simulink model "MicroMouseTemplate"  (R2024a)
settings: Solver=FixedStepAuto  StartTime=0.0  StopTime=2  RelTol=1e-3  EnableMultiTasking=on
undefined symbols (not defined in the file): samplingTime
settings Model: STM32="{\"DigitalPortWrite\":[{\"ID\":\"MicroMouseTemplate:84:3\"},{\"ID\":\"MicroMouseTemplate:84:4\"},{\"ID\":\"MicroMouseTemplate:84:5\"},{\"ID\":\"MicroMouseTemplate:84:6\"},{\"ID\":\"MicroMouseTemplate:84:7\"},{\"ID\":\"MicroMouseTemplate:84:8\"},{\"ID\":\"MicroMouseTemplate:84:9\"},{\"ID\":\"MicroMouseTemplate:84:10\"},{\"ID\":\"MicroMouseTemplate:160:19\"},{\"ID\":\"MicroMouseTemplate:2479:4\"},{\"ID\":\"MicroMouseTemplate:2479:6\"},{\"ID\":\"MicroMouseTemplate:2479:7\"},{\"ID\":\"MicroMouseTemplate:2479:8\"},{\"ID\":\"MicroMouseTemplate1:84:3\"},{\"ID\":\"MicroMouseTemplate1:84:4\"},{\"ID\":\"MicroMouseTemplate1:84:5\"},{\"ID\":\"MicroMouseTemplate1:84:6\"},{\"ID\":\"MicroMouseTemplate1:84:7\"},{\"ID\":\"MicroMouseTemplate1:84:8\"},{\"ID\":\"MicroMouseTemplate1:84:9\"},{\"ID\":\"MicroMouseTemplate1:84:10\"},{\"ID\":\"MicroMouseTemplate1:160:19\"},{\"ID\":\"MicroMouseTemplate1:2479:4\"},{\"ID\":\"MicroMouseTemplate1:2479:6\"},{\"ID\":\"MicroMouseTemplate1:2479:7\"},{\"ID\":\"MicroMouseTemplate1:2479:8\"}],\"PWMOutput\":[{\"ID\":\"MicroMouseTemplate:160:24\"},{\"ID\":\"MicroMouseTemplate:160:25\"},{\"ID\":\"MicroMouseTemplate1:160:24\"},{\"ID\":\"MicroMouseTemplate1:160:25\"}],\"AnalogInput\":[{\"ID\":\"MicroMouseTemplate:2357:1\"},{\"ID\":\"MicroMouseTemplate1:2357:1\"}],\"DigitalPortRead\":[{\"ID\":\"MicroMouseTemplate:2483:3\"},{\"ID\":\"MicroMouseTemplate:2483:4\"},{\"ID\":\"MicroMouseTemplate1:2483:3\"},{\"ID\":\"MicroMouseTemplate1:2483:4\"}]}"  SimulationMode=external  ExtModeTrigDuration=10  Creator=JesseJabezArendse  LastModifiedBy=phila
settings SolverCC: AllowMultiTaskInputOutput=on  AutoInsertRateTranBlk=on  InsertRTBMode=Never (minimum delay)
settings OptimizationCC: EnhancedBackFolding=on  PassReuseOutputArgsAs=Individual arguments  StateBitsets=on  DataBitsets=on  ZeroExternalMemoryAtStartup=off  ZeroInternalMemoryAtStartup=off  NoFixptDivByZeroProtection=on  MaxStackSize=64  OptimizeBlockOrder=speed  DifferentSizesBufferReuse=on  EfficientTunableParamExpr=on
settings DebuggingCC: MultiTaskCondExecSysMsg=none  ParameterOverflowMsg=none  ParameterPrecisionLossMsg=none  ParameterTunabilityLossMsg=error
settings HardwareCC: ProdBitPerPointer=32  ProdBitPerSizeT=32  ProdBitPerPtrDiffT=32  ProdLargestAtomicInteger=Long  ProdLargestAtomicFloat=Double  ProdWordSize=32  ProdLongLongMode=on  ProdHWDeviceType=ARM Compatible->ARM Cortex  TargetBitPerPointer=64  TargetBitPerSizeT=64  TargetBitPerPtrDiffT=64  TargetLongLongMode=on  TargetIntDivRoundTo=Zero  TargetEndianess=LittleEndian  TargetWordSize=64  TargetHWDeviceType=MATLAB Host
settings ModelReferenceCC: EnableParallelModelReferenceBuilds=on  ParallelModelReferenceMATLABWorkerInit=Copy Base Workspace  SupportModelReferenceSimTargetCustomCode=on
settings SFSimCC: MATLABDynamicMemAlloc=off  SimHardwareAcceleration=native
settings RTWCC: Description=Embedded Coder  SystemTargetFile=ert.tlc  HardwareBoard=STM32L4xx Based  TLCOptions=-p0 -aInlineSetEventsForThisBaseRateFcn=TLC_FALSE -aSuppressMultiTaskScheduler=TLC_FALSE -aRateBasedStepFcn=1  TemplateMakefile=ert_default_tmf  Toolchain=GNU Tools for ARM Embedded Processors  CodeExecutionProfiling=on  CodeProfilingInstrumentation=coarse  GPUComputeCapability=3.5
settings RTWCC: CustomHeaderCode=|
  | #include "MicroMouseProgramming\Core\Inc\IMU.h"
  | #include "MicroMouseProgramming\Core\Inc\CustomWhile.h"
  | #include "MicroMouseProgramming\Core\Inc\Motors.h"
settings RTWCC: CustomInclude=|
  | MicroMouseProgramming\Core\Inc\
  | MicroMouseProgramming\Core\Src\
settings RTWCC: CustomSource=|
  | MicroMouseProgramming\Core\Src\IMU.c
  | MicroMouseProgramming\Core\Src\CustomWhile.c
  | MicroMouseProgramming\Core\Src\Motors.c
settings CodeAppCC: ForceParamTrailComments=on  IgnoreCustomStorageClasses=off  OperatorAnnotations=on  SimulinkDataObjDesc=on  SFDataObjDesc=on  InsertBlockDesc=on
settings ERTTargetCC: CodeReplacementLibrary=ARM Cortex-M  SupportNonFinite=off  SupportComplex=off  ExtModeTransport=3  ExtModeStaticAlloc=on  ExtModeStaticAllocSize=2048  ExtModeMexFile=ext_xcp  ExtModeIntrfLevel=Level2 - Open

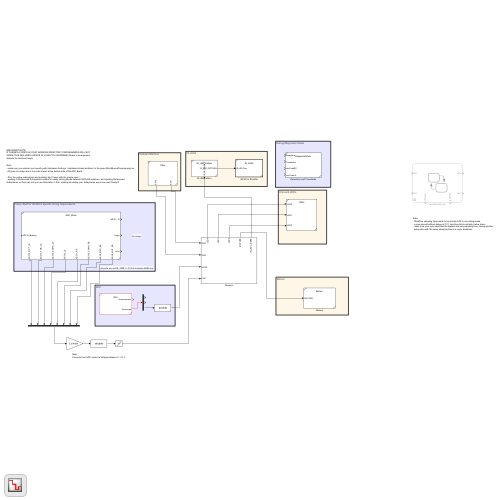
[thumbnail: Simulink's stored preview of the top-level diagram]
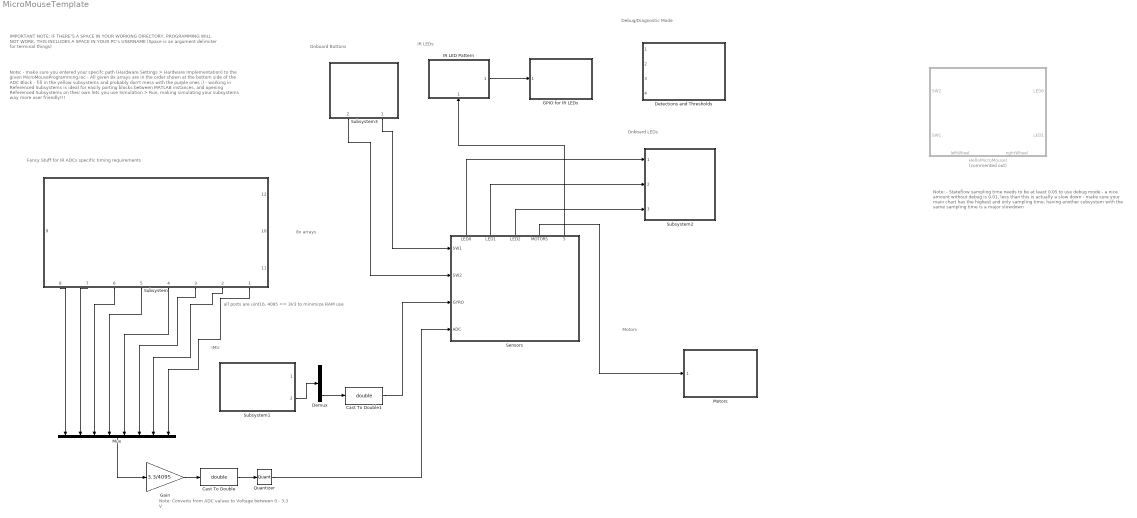
== system MicroMouseTemplate ==
  note: IMPORTANT NOTE:
      | IF THERE'S A SPACE IN YOUR WORKING DIRECTORY, PROGRAMMING WILL NOT WORK, THIS INCLUDES A SPACE IN YOUR PC's USERNAME (Space is an argument delimiter for terminal things)
  note: Note:
      | - make sure you entered your specifc path (Hardware Settings > Hardware Implementation) to the given MicroMouseProgramming.ioc
      | - All given 8x arrays are in the order shown at the bottom side of the ADC Block
      |
      | - fill in the yellow subsystems and probably don't mess with the purple ones :)
      | - working in Referenced Subsystems is ideal for easily porting blocks between MATLAB instances, and opening Referenced Subsystems on their own lets you use Simulation > Run, making simulating your subsystems way more user friendly!!!
  note: 8x arrays
  note: all ports are uint16, 4095 == 3V3 to minimize RAM use
  note: IMU
  note: Note:
      | - Stateflow sampling time needs to be at least 0.05 to use debug mode
      | - a nice amount without debug is 0.01, less than this is actually a slow down
      | - make sure your main chart has the highest and only sampling time, having another
      | subsystem with the same sampling time is a major slowdown
  note: Fancy Stuff for IR ADCs specific timing requirements
  note: IR LEDs
  note: Motors
  note: Onboard Buttons
  note: Onboard LEDs
  note: Debug/Diagnostic Mode
  note: Note:
      | Converts from ADC values to Voltage between 0 - 3.3 V
  Cast To Double : DataTypeConversion  OutDataTypeStr=double  SaturateOnIntegerOverflow=off  RndMeth=Floor
  Cast To Double1 : DataTypeConversion  OutDataTypeStr=double  SaturateOnIntegerOverflow=off  RndMeth=Floor
  Demux : Demux  Outputs=3
  Detections and Thresholds : Subsystem  ReferencedSubsystem=DiagnosticMode
  GPIO for IR LEDs : Subsystem  TreatAsAtomicUnit=on  SystemSampleTime=samplingTime  ReferencedSubsystem=IR_LEDs
  Gain : Gain  Gain=3.3/4095
  HelloMicroMouse! : Stateflow chart  Commented=on  TreatAsAtomicUnit=on
      settings: PortSchema="{\"entries\":[{\"content\":{\"sides\":[{\"content\":{\"connectorIds\":[\"In1\",\"In2\"]},\"type\":\"ConnectorPlacement.EquallySpacedRectSide\",\"uuid\":\"f52daa4f-6374-42e5-9ef1-0ccc99d09b58\"},{\"content\":{\"connectorIds\":[\"Out1\",\"Out2\"],\"side\":\"RIGHT\"},\"type\":\"ConnectorPlacement.EquallySpacedRectSide\",\"uuid\":\"94b478cc-4dde-45c7-a588-77cf2b43cdb7\"},{\"content\":{\"side\":\"TOP\"},\"type\":\"ConnectorPlacement.EquallySpacedRectSide\",\"uuid\":\"afff2079-ea5c-423e-9722-09c3bbce433b\"},{\"content\":{\"connectorIds\":[\"Out3\",\"Out4\"],\"side\":\"BOTTOM\"},\"type\":\"ConnectorPlacement.EquallySpacedRectSide\",\"uuid\":\"94e93a1d-795d-41a3-b2d8-d520b2bf47ef\"}]},\"type\":\"ConnectorPlacement.EquallySpacedConnector\",\"uuid\":\"d4d35636-54af-48ac-af70-d56caef5e090\"}],\"packageUris\":[\"http://schema.mathworks.com/mf0/Connector/R2020b\"],\"version\":\"1.0\"}"
  IR LED Pattern : Subsystem  ReferencedSubsystem=IR_LED_Pattern
      settings: PortSchema="{\"entries\":[{\"content\":{\"sides\":[{\"content\":{},\"type\":\"ConnectorPlacement.EquallySpacedRectSide\",\"uuid\":\"7c8d8a80-aae0-409b-9cb9-b3b86d39018b\"},{\"content\":{\"connectorIds\":[\"Out1\"],\"side\":\"RIGHT\"},\"type\":\"ConnectorPlacement.EquallySpacedRectSide\",\"uuid\":\"c87144cc-2119-421f-99f2-b7a3c226c36e\"},{\"content\":{\"side\":\"TOP\"},\"type\":\"ConnectorPlacement.EquallySpacedRectSide\",\"uuid\":\"a76ebbaf-a86a-4c95-ac8a-0df310e45d39\"},{\"content\":{\"connectorIds\":[\"In1\"],\"side\":\"BOTTOM\"},\"type\":\"ConnectorPlacement.EquallySpacedRectSide\",\"uuid\":\"3df1aa50-ad1c-403c-a4a5-6da959ac349c\"}]},\"type\":\"ConnectorPlacement.EquallySpacedConnector\",\"uuid\":\"b655e760-2cb2-4645-8a40-e85195c99b66\"}],\"packageUris\":[\"http://schema.mathworks.com/mf0/Connector/R2020b\"],\"version\":\"1.0\"}"
  Motors : Subsystem  ReferencedSubsystem=Motors
  Mux : Mux  Inputs=8
  Quantizer : Quantizer  QuantizationInterval=0.01
  Sensors : Subsystem
      settings: PortSchema="{\"entries\":[{\"content\":{\"sides\":[{\"content\":{\"connectorIds\":[\"In1\",\"In2\",\"In3\",\"In4\"]},\"type\":\"ConnectorPlacement.EquallySpacedRectSide\",\"uuid\":\"bc6db5eb-46dc-4f8e-8cde-60f150010aca\"},{\"content\":{\"side\":\"RIGHT\"},\"type\":\"ConnectorPlacement.EquallySpacedRectSide\",\"uuid\":\"e71d750a-c6fe-4d02-b611-1eb45a9e699c\"},{\"content\":{\"connectorIds\":[\"Out1\",\"Out2\",\"Out3\",\"Out4\",\"Out5\"],\"side\":\"TOP\"},\"type\":\"ConnectorPlacement.EquallySpacedRectSide\",\"uuid\":\"16229a75-dc4c-4034-8ad6-a6d33f431b7e\"},{\"content\":{\"side\":\"BOTTOM\"},\"type\":\"ConnectorPlacement.EquallySpacedRectSide\",\"uuid\":\"378b0be1-cc28-458e-984c-d88580dc795a\"}]},\"type\":\"ConnectorPlacement.EquallySpacedConnector\",\"uuid\":\"81c8b409-cb86-489b-9c0e-9f4aaa37c54e\"}],\"packageUris\":[\"http://schema.mathworks.com/mf0/Connector/R2020b\"],\"version\":\"1.0\"}"
  Subsystem : Subsystem  ReferencedSubsystem=ADC_Block
      settings: PortSchema="{\"entries\":[{\"content\":{\"sides\":[{\"content\":{},\"type\":\"ConnectorPlacement.EquallySpacedRectSide\",\"uuid\":\"be6b81d5-7a49-4e34-b35f-0c07892094fc\"},{\"content\":{\"connectorIds\":[\"Out1\",\"Out2\",\"Out3\",\"Out4\",\"Out5\",\"Out6\",\"Out7\",\"Out8\"],\"side\":\"RIGHT\"},\"type\":\"ConnectorPlacement.EquallySpacedRectSide\",\"uuid\":\"5e22590a-b7c0-4c63-8de4-8d81fd6c3849\"},{\"content\":{\"connectorIds\":[\"Out12\",\"Out10\",\"Out11\"],\"side\":\"TOP\"},\"type\":\"ConnectorPlacement.EquallySpacedRectSide\",\"uuid\":\"da97636e-cea0-4a10-8fe5-d807f9ee999f\"},{\"content\":{\"connectorIds\":[\"Out9\"],\"side\":\"BOTTOM\"},\"type\":\"ConnectorPlacement.EquallySpacedRectSide\",\"uuid\":\"a593d780-81a8-4730-a8bc-2bbf356cafe4\"}]},\"type\":\"ConnectorPlacement.EquallySpacedConnector\",\"uuid\":\"0bcac921-e51a-4437-9183-315712d0a8c2\"}],\"packageUris\":[\"http://schema.mathworks.com/mf0/Connector/R2020b\"],\"version\":\"1.0\"}"
  Subsystem1 : Subsystem  ReferencedSubsystem=IMU
  Subsystem2 : Subsystem  ReferencedSubsystem=LEDs
  Subsystem3 : Subsystem  ReferencedSubsystem=SWs
      settings: PortSchema="{\"entries\":[{\"content\":{\"sides\":[{\"content\":{},\"type\":\"ConnectorPlacement.EquallySpacedRectSide\",\"uuid\":\"e28eebbe-b7f2-4b36-b777-f04b3fc0ab34\"},{\"content\":{\"side\":\"RIGHT\"},\"type\":\"ConnectorPlacement.EquallySpacedRectSide\",\"uuid\":\"8c3fa4f5-1e6a-4f41-8e39-119bdbcbe036\"},{\"content\":{\"side\":\"TOP\"},\"type\":\"ConnectorPlacement.EquallySpacedRectSide\",\"uuid\":\"44ec265b-fcc9-41a2-b2aa-224ec14b1e13\"},{\"content\":{\"connectorIds\":[\"Out2\",\"Out1\"],\"side\":\"BOTTOM\"},\"type\":\"ConnectorPlacement.EquallySpacedRectSide\",\"uuid\":\"b53c205f-8dfa-45db-b859-d3829686a648\"}]},\"type\":\"ConnectorPlacement.EquallySpacedConnector\",\"uuid\":\"83ae30f7-f6c1-458e-af88-9bb28644e581\"}],\"packageUris\":[\"http://schema.mathworks.com/mf0/Connector/R2020b\"],\"version\":\"1.0\"}"
  wires:
  IR LED Pattern/1 -> GPIO for IR LEDs/1
  Subsystem/2 -> Mux/7
  Subsystem/7 -> Mux/2
  Subsystem3/1 -> Sensors/1(SW1)
  Subsystem3/2 -> Sensors/2(SW2)
  Sensors/4(MOTORS) -> Motors/1
  Sensors/1(LED0) -> Subsystem2/1
  Subsystem/4 -> Mux/5
  Subsystem/5 -> Mux/4
  Subsystem/1 -> Mux/8
  Subsystem/3 -> Mux/6
  Subsystem/8 -> Mux/1
  Subsystem/6 -> Mux/3
  Quantizer/1 -> Sensors/4(ADC)
  Sensors/2(LED1) -> Subsystem2/2
  Sensors/3(LED2) -> Subsystem2/3
  Mux/1 -> Gain/1
  Cast To Double/1 -> Quantizer/1
  Gain/1 -> Cast To Double/1
  Sensors/5(IR_LEDs_SIDES) -> IR LED Pattern/1
  Demux/3 -> Cast To Double1/1
  Subsystem1/2 -> Demux/1
  Cast To Double1/1 -> Sensors/3(GYRO)

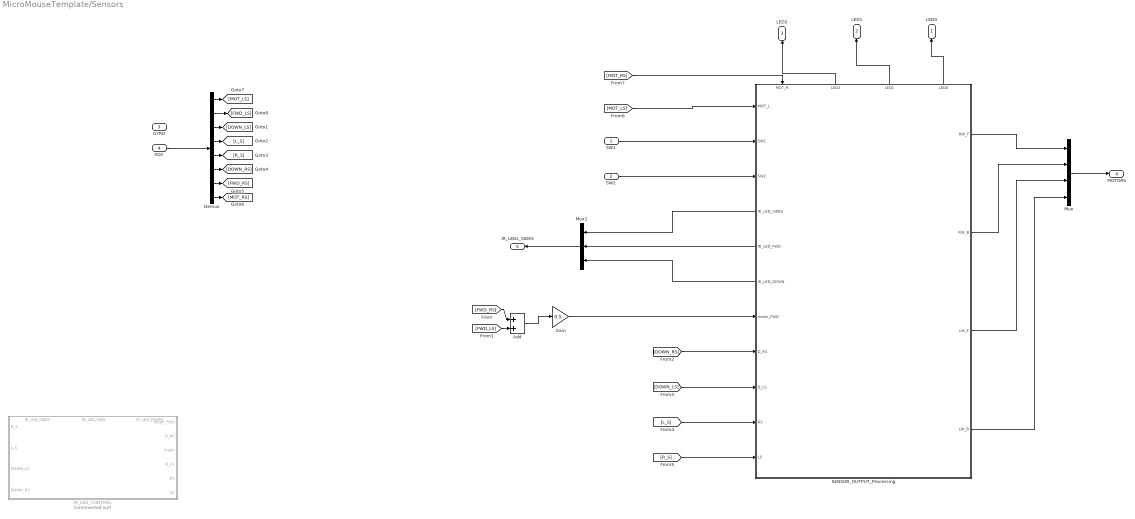
== system MicroMouseTemplate/Sensors ==
  SW1 : Inport
  SW2 : Inport  Port=2
  GYRO : Inport  Port=3
  ADC : Inport  Port=4
  Add : Sum
  Demux : Demux  Outputs=8
  Gain : Gain  Gain=0.5
  IR_LED_CONTROL : Stateflow chart  Commented=on  TreatAsAtomicUnit=on
      settings: PortSchema="{\"entries\":[{\"content\":{\"sides\":[{\"content\":{\"connectorIds\":[\"In2\",\"In3\",\"In5\",\"In4\"]},\"type\":\"ConnectorPlacement.EquallySpacedRectSide\",\"uuid\":\"6ddea5f0-ded9-4726-b8e4-d6f2d38f9761\"},{\"content\":{\"connectorIds\":[\"Out1\",\"Out2\",\"In1\",\"Out3\",\"Out4\",\"Out5\"],\"side\":\"RIGHT\"},\"type\":\"ConnectorPlacement.EquallySpacedRectSide\",\"uuid\":\"6b06b77d-6c18-44e2-b7ed-08393e6b8e65\"},{\"content\":{\"connectorIds\":[\"Out8\",\"Out7\",\"Out6\"],\"side\":\"TOP\"},\"type\":\"ConnectorPlacement.EquallySpacedRectSide\",\"uuid\":\"b6a40ded-61fd-4c1c-a30f-2796126667e7\"},{\"content\":{\"side\":\"BOTTOM\"},\"type\":\"ConnectorPlacement.EquallySpacedRectSide\",\"uuid\":\"f6f9d052-d44c-4dc6-9c48-54afbab78fdb\"}]},\"type\":\"ConnectorPlacement.EquallySpacedConnector\",\"uuid\":\"44f3d40a-ac67-4a28-8278-d7359b0b7d12\"}],\"packageUris\":[\"http://schema.mathworks.com/mf0/Connector/R2020b\"],\"version\":\"1.0\"}"
  Mux : Mux
  Mux1 : Mux  Inputs=3
  SENSOR_OUTPUT_Processing : Stateflow chart  TreatAsAtomicUnit=on
      settings: PortSchema="{\"entries\":[{\"content\":{\"sides\":[{\"content\":{\"connectorIds\":[\"In2\",\"In3\",\"In4\",\"Out3\",\"Out2\",\"Out1\",\"In5\",\"In9\",\"In8\",\"In6\",\"In7\"]},\"type\":\"ConnectorPlacement.EquallySpacedRectSide\",\"uuid\":\"a9fa26fe-b8b4-44a7-ba43-f236deb27886\"},{\"content\":{\"connectorIds\":[\"Out5\",\"Out6\",\"Out7\",\"Out8\"],\"side\":\"RIGHT\"},\"type\":\"ConnectorPlacement.EquallySpacedRectSide\",\"uuid\":\"821e32f5-16df-4623-bfe7-25c75d2fd732\"},{\"content\":{\"connectorIds\":[\"In1\",\"Out9\",\"Out10\",\"Out4\"],\"side\":\"TOP\"},\"type\":\"ConnectorPlacement.EquallySpacedRectSide\",\"uuid\":\"5c28d776-49d7-4147-b157-b96caf1d4972\"}]},\"type\":\"ConnectorPlacement.EquallySpacedConnector\",\"uuid\":\"32d8ea96-50da-4ded-ba61-48993f917b2f\"}],\"packageUris\":[\"http://schema.mathworks.com/mf0/Connector/R2020b\"],\"version\":\"1.0\"}"
  LED0 : Outport
  LED1 : Outport  Port=2
  LED2 : Outport  Port=3
  MOTORS : Outport  Port=4
  IR_LEDs_SIDES : Outport  Port=5
  wires:
  Add/1 -> Gain/1
  SENSOR_OUTPUT_Processing/4(LED0) -> LED0/1
  SENSOR_OUTPUT_Processing/5(RW_F) -> Mux/1
  SENSOR_OUTPUT_Processing/6(RW_B) -> Mux/2
  SENSOR_OUTPUT_Processing/7(LW_F) -> Mux/3
  SENSOR_OUTPUT_Processing/8(LW_B) -> Mux/4
  SW1/1 -> SENSOR_OUTPUT_Processing/3(SW1)
  SW2/1 -> SENSOR_OUTPUT_Processing/4(SW2)
  ADC/1 -> Demux/1
  Demux/1 -> [MOT_LS]
  Demux/6 -> [DOWN_RS]
  Demux/8 -> [MOT_RS]
  Demux/3 -> [DOWN_LS]
  Demux/2 -> [FWD_LS]
  Demux/4 -> [L_S]
  Demux/5 -> [R_S]
  Demux/7 -> [FWD_RS]
  [FWD_RS] -> Add/1
  [FWD_LS] -> Add/2
  Mux/1 -> MOTORS/1
  SENSOR_OUTPUT_Processing/10(LED1) -> LED1/1
  SENSOR_OUTPUT_Processing/9(LED2) -> LED2/1
  Gain/1 -> SENSOR_OUTPUT_Processing/5(mean_FWD)
  Mux1/1 -> IR_LEDs_SIDES/1
  SENSOR_OUTPUT_Processing/1(IR_LED_DOWN) -> Mux1/3
  [L_S] -> SENSOR_OUTPUT_Processing/6(RS)
  [R_S] -> SENSOR_OUTPUT_Processing/7(LS)
  [DOWN_RS] -> SENSOR_OUTPUT_Processing/9(D_RS)
  [DOWN_LS] -> SENSOR_OUTPUT_Processing/8(D_LS)
  SENSOR_OUTPUT_Processing/3(IR_LED_SIDES) -> Mux1/1
  SENSOR_OUTPUT_Processing/2(IR_LED_FWD) -> Mux1/2
  [MOT_LS] -> SENSOR_OUTPUT_Processing/2(MOT_L)
  [MOT_RS] -> SENSOR_OUTPUT_Processing/1(MOT_R)

== stateflow chart MicroMouseTemplate/HelloMicroMouse! ==
  state ButtonPressed
    entry:
    LED0 = true;
    LED1 = true;
    state Right
      entry:
      leftWheel = 80;
      rightWheel = 80;
    state Left
      entry:
      leftWheel = 80;
      rightWheel = 80;
    (default) -> Left
    Left -> Right : after(0.5,sec)
    Right -> Left : after(0.5,sec)
  state Stop
    entry:
    LED0 = false;
    LED1 = false;
    leftWheel = 0;
    rightWheel = 0;
  state WaitUntilButtonPressed
    during:
    LED0 = ~LED0;
  (default) -> WaitUntilButtonPressed
  ButtonPressed -> Stop : [SW2]
  WaitUntilButtonPressed -> ButtonPressed : [SW1]
  data: SW2 input; LED0 output; LED1 output; SW1 input; leftWheel output int8; rightWheel output int8

== stateflow chart MicroMouseTemplate/Sensors/SENSOR_OUTPUT_Processing ==
  state ON_MODE
    entry:
    LED0 = true;
    state Line_Following
      entry:
      LED0 = false;
      LED1 = false;
      during:
      error = double(D_LS) - double(D_RS);
      error = error*100/3.3;
      LW_F = 79.5 - error*0.4;
      RW_F = 80 +error*0.4;
    state Stop
      entry:
      LED0 = false;
      LW_F = 0;
      RW_F = 0;
      LW_B = 0;
      RW_B = 0;
    state U_Turn
      entry:
      GOAL_R = 0;
      GOAL_L = 0;
      during:
      LED1 = ~LED1;
      RW_F = 90;
      LW_B = 90;
    state CalibrateOTHER
      entry:
      IR_LED_FWD = 1;
      IR_LED_SIDES = 0;
      IR_LED_DOWN = 1;
      during:
      FWD_Threshold = mean_FWD*0.8;
      DOWN_RS_Threshold = D_RS;
      DOWN_LS_Threshold = D_LS;
      exit:
      IR_LED_FWD = 1;
      IR_LED_SIDES = 0;
      IR_LED_DOWN = 1;
    state CalibrateSIDES
      entry:
      IR_LED_FWD = 0;
      IR_LED_SIDES = 1;
      during:
      LED0 = ~LED0;
      LED2 = ~LED2;
      RS_Threshold = RS*0.95;
      LS_Threshold = LS*0.8;
      exit:
      IR_LED_FWD = 1;
      IR_LED_SIDES = 0;
    state WAIT
    state Initialise
      entry:
      IR_LED_DOWN = 1;
      IR_LED_FWD = 1;
      IR_LED_SIDES = 0;
      LED0 = false;
      LED1 = false;
      LED2 = false;
      GOAL_R = 0;
      GOAL_L = 0;
    state Intersection
      during:
      error = double(D_LS) - double(D_RS);
      error = error*100/3.3;
      LW_F = 80 - error*0.4;
      RW_F = 80 +error*0.4;
      exit:;
      LW_F = 0;
      RW_F = 0;
    state Detect_Sides
      entry:
      FWD_Wall = (mean_FWD > FWD_Threshold);
      IR_LED_FWD = 0;
      IR_LED_SIDES = 1;
      during:
      RIGHT_Wall = (RS > RS_Threshold);
      LEFT_Wall = (LS > LS_Threshold) ;
      exit:
      IR_LED_FWD = 1;
      IR_LED_SIDES = 0;
    state Wall_F
    state TurnR
      entry:
      GOAL_R = GOAL_R +1;
      during:
      LED2 = ~LED2;
      RW_B = 90;
      LW_F = 90;
    state TurnL
      entry:
      GOAL_L = GOAL_L +1;
      during:
      LED0 = ~LED0;
      RW_F = 90;
      LW_B = 90;
    state U_TURN_CALIBRATION
      entry:
      during:
      LED1 = ~LED1;
      RW_F = 90;
      LW_B = 90;
      exit:
      LED1 = false;
      RW_F = 0;
      LW_B = 0
    state R_OR_L
    state No_Turn
      entry:
      GOAL_R = 0;
      GOAL_L = 0;
    state Correction
      during:
      error = double(D_LS) - double(D_RS);
      error = error*100/3.3;
      LW_F = 79.5 - error*0.16;
      RW_F = 80 +error*0.16;
    state Return
      entry:
      LW_F = 0;
      RW_F = 0;
      LW_B = 0;
      RW_B = 0
      FINISH = (GOAL_R ==3) | (GOAL_L == 3);
      FWD_Wall=false;
      RIGHT_Wall =false;
      LEFT_Wall=false;
      LED0 = false;
      LED1 = false;
      LED2 = false;
    state Test_FWD [commented out]
      during:
      FWD_Wall = (mean_FWD > FWD_Threshold);
      if FWD_Wall
      LED1 = true;
      else
      LED1 = false;
      end
    state Test_sides [commented out]
      FWD_Wall = (mean_FWD > FWD_Threshold);
      IR_LED_FWD = 0;
      IR_LED_SIDES = 1;
      during:
      RIGHT_Wall = (RS > RS_Threshold);
      if RIGHT_Wall
      LED2 = true;
      else
      LED2 = false;
      end
      LEFT_Wall = (LS > LS_Threshold) ;
      if LEFT_Wall
      LED0 = true;
      else
      LED0 = false;
      end
      exit:
      IR_LED_FWD = 1;
      IR_LED_SIDES = 0
    state FINISH
      entry:
      LED0 = true;
      LED1 = false;
      LED2 = true;
      during:
      LED0 = ~LED0;
      LED1 = ~LED1;
      LED2 = ~LED2;
      exit:
      LED0 = false;
      LED1 = false;
      LED2 = false;
    state Spin_L
      during:
      RW_F = 90;
      LW_B = 90;
    state Spin_R
      during:
      RW_B = 90;
      LW_F = 90;
      exit:
      RW_B = 0;
      LW_F = 0;
    state RUN_Done
      entry:
      RW_F = 0;
      LW_B = 0;
      LED0 = false;
      LED1 = false;
      LED2 = false;
    Stop -> WAIT : [SW1]
    (default) -> Initialise
    Line_Following -> Stop [order 1] : [SW2]
    WAIT -> Line_Following [order 1] : [SW1]
    Wall_F -> U_Turn [order 3] : [RIGHT_Wall && LEFT_Wall]
    U_Turn -> Return : after(1.03,sec)
    CalibrateOTHER -> WAIT : after(0.3,sec)
    Initialise -> CalibrateSIDES : [SW2 ]
    U_TURN_CALIBRATION -> WAIT : after(1.06,sec)
    WAIT -> U_TURN_CALIBRATION [order 2] : [SW2]
    RUN_Done -> WAIT : after(0.2,sec)
    CalibrateSIDES -> CalibrateOTHER : [after(0.3,sec)]
    Intersection -> Detect_Sides : [MOT_L >3.25 && MOT_R >3.25]
    Detect_Sides -> Wall_F [order 1] : [FWD_Wall && after(0.2,sec)]
    Wall_F -> TurnR [order 1] : [~RIGHT_Wall && LEFT_Wall]
    Line_Following -> Intersection [order 2] : [MOT_L <3.25 && MOT_R <3.25]
    Wall_F -> TurnL [order 2] : [RIGHT_Wall && ~LEFT_Wall]
    Wall_F -> R_OR_L [order 4] : [~RIGHT_Wall && ~LEFT_Wall]
    TurnR -> Return : after(0.502,sec)
    Detect_Sides -> No_Turn [order 2] : [~FWD_Wall && after(0.2,sec)]
    R_OR_L -> TurnL : after(0.1,sec)
    Correction -> Line_Following : after(0.8,sec)
    TurnL -> Return : after(0.502,sec)
    Return -> Correction [order 2] : [after(0.05,sec)]
    No_Turn -> Return : after(0.1,sec)
    Return -> FINISH [order 1] : [FINISH]
    FINISH -> Spin_R : after(0.2,sec)
    Spin_R -> Spin_L : after(1.1,sec)
    Spin_L -> RUN_Done : after(1.1,sec)
  state START
    entry:
    LED0 = true;
    LED1 = true;
    LED2 = true;
  (default) -> START
  START -> ON_MODE : [SW1]
  data: IR_LED_DOWN output; IR_LED_FWD output; IR_LED_SIDES output; MOT_R input; MOT_L input; SW1 input; SW2 input; mean_FWD input; LED0 output; RW_F output; RW_B output; LW_F output; LW_B output; LED2 output; LED1 output; RS input; LS input; D_LS input; D_RS input; RS_Threshold local; LS_Threshold local; DOWN_RS_Threshold local; DOWN_LS_Threshold local; FWD_Threshold local; error local; RIGHT_Wall local; LEFT_Wall local; FWD_Wall local; FINISH local; GOAL_L local; GOAL_R local

== stateflow chart MicroMouseTemplate/Sensors/IR_LED_CONTROL ==
  state Catpture_mean_FWD
    entry:
    IR_LED_FWD = 1;
    during:
    mean_FWD = mean;
    exit:
    IR_LED_FWD =0 ;
  state Capture_Sides
    entry:
    IR_LED_SIDES = 1;
    during:
    RS = R_S;
    LS = L_S;
    exit:
    IR_LED_SIDES = 0;
  state Capture_down
    entry:
    IR_LED_DOWN = 1;
    during:
    D_RS = DOWN_RS;
    D_LS = DOWN_LS;
    %MOT_L=MOT_LS;
    %MOT_R=MOT_RS;
    exit:
    IR_LED_DOWN = 0;
  (default) -> Catpture_mean_FWD
  Capture_Sides -> Catpture_mean_FWD : after(0.2,sec)
  Catpture_mean_FWD -> Capture_down : after(0.2,sec)
  Capture_down -> Capture_Sides : after(0.2,sec)
  data: mean_FWD output; mean input; R_S input; L_S input; DOWN_RS input; DOWN_LS input; D_RS output; D_LS output; RS output; LS output; IR_LED_DOWN output; IR_LED_FWD output; IR_LED_SIDES output
